simulink model "Magnetic_Levitation_Part3"  (R2022b)
settings: Solver=VariableStepAuto  StartTime=0.0  StopTime=10  RelTol=1e-3
settings Model: Creator=mhadi  LastModifiedBy=mhadi

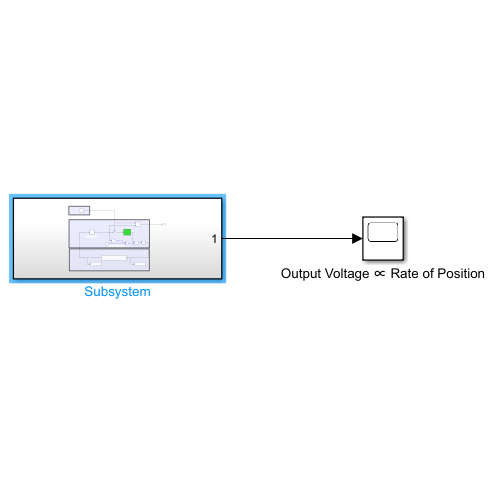
[thumbnail: Simulink's stored preview of the top-level diagram]
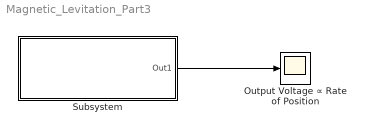
== system Magnetic_Levitation_Part3 ==
  Output Voltage ∝ Rate of Position : Scope
  Subsystem : Subsystem
  wires:
  Subsystem/1(Out1) -> Output Voltage ∝ Rate of Position/1

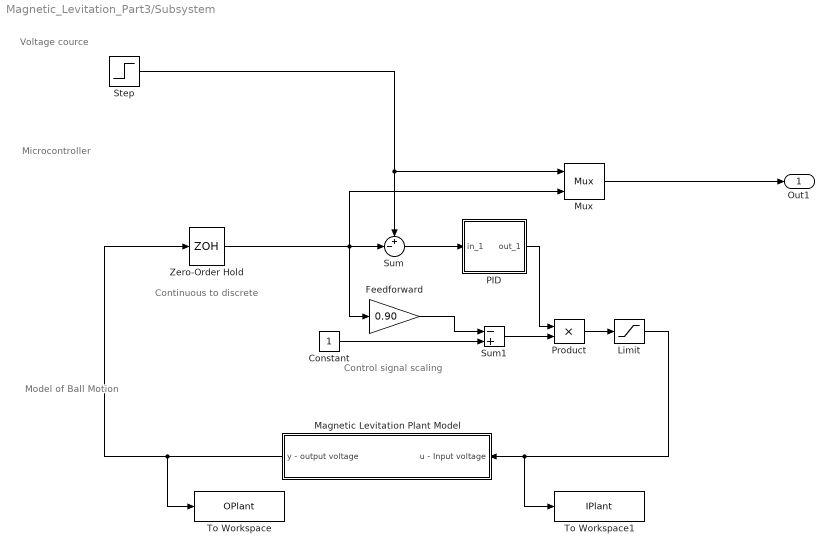
== system Magnetic_Levitation_Part3/Subsystem ==
  note: Voltage cource
  note: Model of Ball Motion
  note: Control signal scaling
  note: Continuous to discrete
  note: Microcontroller
  Constant : Constant  StatePerturbationForJacobian=1.0e-05
  Feedforward : Gain  StatePerturbationForJacobian=1.0e-05  Gain=0.90  SaturateOnIntegerOverflow=on  OutDataTypeStr=Inherit: Same as input  ParamDataTypeStr=Inherit: Same as input
  Limit : Saturate  StatePerturbationForJacobian=1.0e-05  UpperLimit=1  LowerLimit=0  ZeroCross=off
  Magnetic Levitation Plant Model : Subsystem  StatePerturbationForJacobian=1.0e-05
  Mux : Mux  StatePerturbationForJacobian=1.0e-05  Inputs=2
  PID : Subsystem  StatePerturbationForJacobian=1.0e-05  mask(PID){Kp=0.5, Ki=3, Kd=0, Ts=0.001}
      mask prompts: Ts "Sample time:"
      mask help: Discrete-time PID controller with limited integrator
      mask Display: disp('PID');
  Product : Product  StatePerturbationForJacobian=1.0e-05  InputSameDT=on  SaturateOnIntegerOverflow=on  OutDataTypeStr=Inherit: Same as first input
  Step : Step  StatePerturbationForJacobian=1.0e-05  Time=0  SampleTime=0
  Sum : Sum  StatePerturbationForJacobian=1.0e-05  Inputs=+-|  InputSameDT=on  SaturateOnIntegerOverflow=on  OutDataTypeStr=Inherit: Same as first input
  Sum1 : Sum  StatePerturbationForJacobian=1.0e-05  Inputs=-+  InputSameDT=on  SaturateOnIntegerOverflow=on  OutDataTypeStr=Inherit: Same as first input
  To Workspace : ToWorkspace  VariableName=OPlant  SaveFormat=Structure With Time  SampleTime=-1
      settings: Save2DSignal=2-D array (concatenate along first dimension)
  To Workspace1 : ToWorkspace  VariableName=IPlant  SaveFormat=Structure With Time  SampleTime=-1
      settings: Save2DSignal=2-D array (concatenate along first dimension)
  Zero-Order Hold : ZeroOrderHold  StatePerturbationForJacobian=1.0e-05  SampleTime=0.001
  Out1 : Outport
  wires:
  Limit/1 -> To Workspace1/1, Magnetic Levitation Plant Model/1(u - Input voltage)
  PID/1(out_1) -> Product/1
  Sum/1 -> PID/1(in_1)
  Feedforward/1 -> Sum1/1
  Mux/1 -> Out1/1
  Product/1 -> Limit/1
  Zero-Order Hold/1 -> Mux/2, Sum/2, Feedforward/1
  Magnetic Levitation Plant Model/1(y - output voltage) -> To Workspace/1, Zero-Order Hold/1
  Sum1/1 -> Product/2
  Constant/1 -> Sum1/2
  Step/1 -> Mux/1, Sum/1

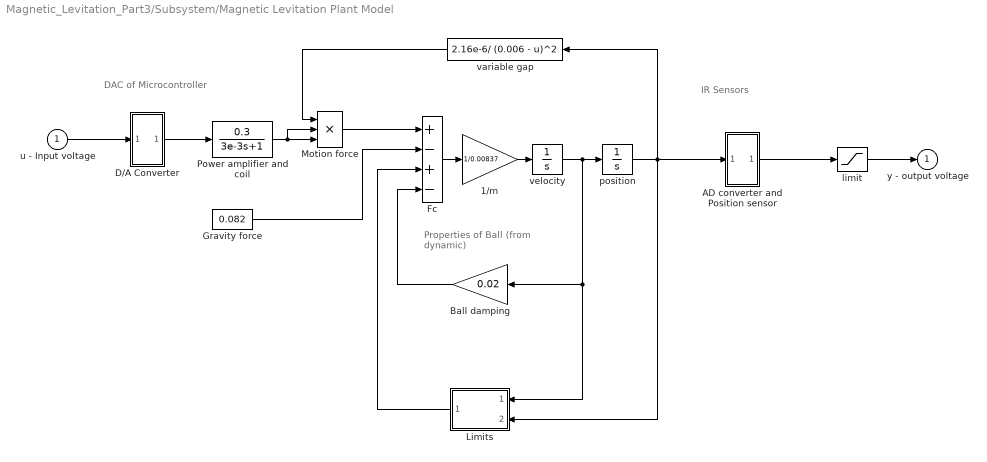
== system Magnetic_Levitation_Part3/Subsystem/Magnetic Levitation Plant Model ==
  note: Properties of Ball
      | (from dynamic)
  note: IR Sensors
  note: DAC of
      | Microcontroller
  u - Input voltage : Inport  StatePerturbationForJacobian=1.0e-05
  " limit" : Saturate  StatePerturbationForJacobian=1.0e-05  UpperLimit=0.998  LowerLimit=0  ZeroCross=off
  1/m : Gain  StatePerturbationForJacobian=1.0e-05  Gain=1/0.00837  SaturateOnIntegerOverflow=on  OutDataTypeStr=Inherit: Same as input  ParamDataTypeStr=Inherit: Same as input
  AD converter and Position sensor : Subsystem  StatePerturbationForJacobian=1.0e-05
      mask Display: disp('A/D')
  Ball damping : Gain  StatePerturbationForJacobian=1.0e-05  Gain=0.02  SaturateOnIntegerOverflow=on  OutDataTypeStr=Inherit: Same as input  ParamDataTypeStr=Inherit: Same as input
  D/A Converter : Subsystem  StatePerturbationForJacobian=1.0e-05
      mask Display: disp('D/A')
  Fc : Sum  StatePerturbationForJacobian=1.0e-05  Inputs=+-+-  InputSameDT=on  SaturateOnIntegerOverflow=on  OutDataTypeStr=Inherit: Same as first input
  Gravity force : Constant  StatePerturbationForJacobian=1.0e-05  Value=0.082
  Limits : Subsystem  StatePerturbationForJacobian=1.0e-05
      mask Display: disp('LIMIT')
  Motion force : Product  StatePerturbationForJacobian=1.0e-05  Inputs=3  InputSameDT=on  SaturateOnIntegerOverflow=on  OutDataTypeStr=Inherit: Same as first input
  Power amplifier and coil : TransferFcn  StatePerturbationForJacobian=1.0e-05  Numerator=[0.3]  Denominator=[3e-3 1]
  position : Integrator  StatePerturbationForJacobian=1.0e-05  LimitOutput=on  UpperSaturationLimit=0.005  LowerSaturationLimit=0  ZeroCross=off
  variable gap : Fcn  StatePerturbationForJacobian=1.0e-05  Expr=2.16e-6/ (0.006 - u)^2
  velocity : Integrator  StatePerturbationForJacobian=1.0e-05  ZeroCross=off
  y - output voltage : Outport  StatePerturbationForJacobian=1.0e-05
  wires:
  velocity/1 -> Ball damping/1, Limits/1(velocity), position/1
  Ball damping/1 -> Fc/4
  variable gap/1 -> Motion force/1
  1/m/1 -> velocity/1
  Fc/1 -> 1/m/1
  Motion force/1 -> Fc/1
  Gravity force/1 -> Fc/2
  D/A Converter/1(out_1) -> Power amplifier and coil/1
  u - Input voltage/1 -> D/A Converter/1(in_1)
  position/1 -> AD converter and Position sensor/1(in_1), variable gap/1, Limits/2(position)
  Limits/1(force) -> Fc/3
  Power amplifier and coil/1 -> Motion force/3, Motion force/2
  " limit"/1 -> y - output voltage/1
  AD converter and Position sensor/1(out_1) -> " limit"/1

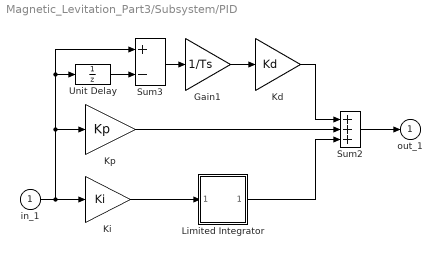
== system Magnetic_Levitation_Part3/Subsystem/PID ==
  in_1 : Inport  StatePerturbationForJacobian=1.0e-05
  Gain1 : Gain  StatePerturbationForJacobian=1.0e-05  Gain=1/Ts  SaturateOnIntegerOverflow=on  OutDataTypeStr=Inherit: Same as input  ParamDataTypeStr=Inherit: Same as input
  Kd : Gain  StatePerturbationForJacobian=1.0e-05  Gain=Kd  SaturateOnIntegerOverflow=on  OutDataTypeStr=Inherit: Same as input  ParamDataTypeStr=Inherit: Same as input
  Ki : Gain  StatePerturbationForJacobian=1.0e-05  Gain=Ki  SaturateOnIntegerOverflow=on  OutDataTypeStr=Inherit: Same as input  ParamDataTypeStr=Inherit: Same as input
  Kp : Gain  StatePerturbationForJacobian=1.0e-05  Gain=Kp  SaturateOnIntegerOverflow=on  OutDataTypeStr=Inherit: Same as input  ParamDataTypeStr=Inherit: Same as input
  Limited Integrator : Subsystem  StatePerturbationForJacobian=1.0e-05  mask(Discrete-Time Limited Integrator.){lower_limit=0, upper_limit=2, X0=0, Ts=Ts}
      mask prompts: lower_limit "Lower bound:"; upper_limit "Upper bound:"; X0 "Initial condition:"; Ts "Sampling Time:"
      mask help: Discrete-Time Limited Integrator.
      mask Help: Discrete-Time Limited Integrator. Unmask to see details.
      mask Display: plot(-1,-0.2,3.5,1.2,[0,1,2,2.9],[0,0,1,1],[0,1],[0.5,0.5], [.5,.5], [.8,.6], [.05,.35,.05,.35],[.4,.4,.2,.2], [.45,.65],[.3,.3], [.9,.9],[.2,.4]);
  Sum2 : Sum  StatePerturbationForJacobian=1.0e-05  Inputs=+++  InputSameDT=on  SaturateOnIntegerOverflow=on  OutDataTypeStr=Inherit: Same as first input
  Sum3 : Sum  StatePerturbationForJacobian=1.0e-05  Inputs=+-  InputSameDT=on  SaturateOnIntegerOverflow=on  OutDataTypeStr=Inherit: Same as first input
  Unit Delay : UnitDelay  StatePerturbationForJacobian=1.0e-05  SampleTime=Ts  HasFrameUpgradeWarning=on
  out_1 : Outport  StatePerturbationForJacobian=1.0e-05  InitialOutput=0
  wires:
  Unit Delay/1 -> Sum3/2
  Kd/1 -> Sum2/1
  Kp/1 -> Sum2/2
  Sum2/1 -> out_1/1
  Sum3/1 -> Gain1/1
  Gain1/1 -> Kd/1
  in_1/1 -> Ki/1, Sum3/1, Unit Delay/1, Kp/1
  Ki/1 -> Limited Integrator/1(in_1)
  Limited Integrator/1(out_1) -> Sum2/3

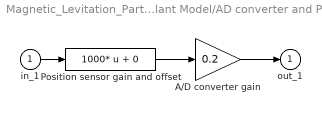
== system Magnetic_Levitation_Part3/Subsystem/Magnetic Levitation Plant Model/AD converter and Position sensor ==
  in_1 : Inport  StatePerturbationForJacobian=1.0e-05
  A/D converter gain : Gain  StatePerturbationForJacobian=1.0e-05  Gain=0.2  SaturateOnIntegerOverflow=on  OutDataTypeStr=Inherit: Same as input  ParamDataTypeStr=Inherit: Same as input
  Position sensor gain and offset : Fcn  StatePerturbationForJacobian=1.0e-05  Expr=1000* u + 0
  out_1 : Outport  StatePerturbationForJacobian=1.0e-05
  wires:
  in_1/1 -> Position sensor gain and offset/1
  Position sensor gain and offset/1 -> A/D converter gain/1
  A/D converter gain/1 -> out_1/1

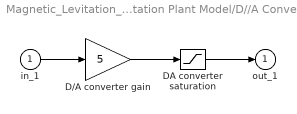
== system Magnetic_Levitation_Part3/Subsystem/Magnetic Levitation Plant Model/D//A Converter ==
  in_1 : Inport  StatePerturbationForJacobian=1.0e-05
  D/A converter gain : Gain  StatePerturbationForJacobian=1.0e-05  Gain=5  SaturateOnIntegerOverflow=on  OutDataTypeStr=Inherit: Same as input  ParamDataTypeStr=Inherit: Same as input
  DA converter saturation : Saturate  StatePerturbationForJacobian=1.0e-05  UpperLimit=5  LowerLimit=-5  ZeroCross=off
  out_1 : Outport  StatePerturbationForJacobian=1.0e-05
  wires:
  in_1/1 -> D/A converter gain/1
  DA converter saturation/1 -> out_1/1
  D/A converter gain/1 -> DA converter saturation/1

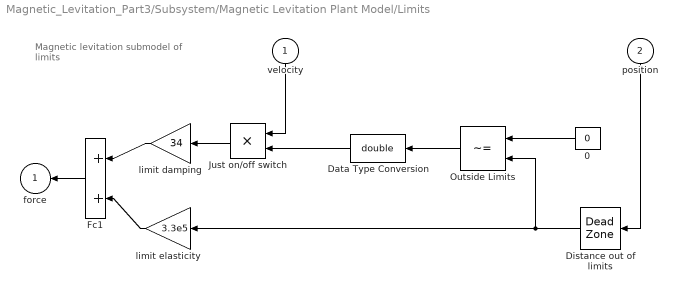
== system Magnetic_Levitation_Part3/Subsystem/Magnetic Levitation Plant Model/Limits ==
  note: Magnetic levitation
      | submodel of limits
  velocity : Inport  StatePerturbationForJacobian=1.0e-05
  position : Inport  StatePerturbationForJacobian=1.0e-05  Port=2
  0 : Constant  StatePerturbationForJacobian=1.0e-05  Value=0
  Data Type Conversion : DataTypeConversion  StatePerturbationForJacobian=1.0e-05  OutDataTypeStr=double
  Distance out of limits : DeadZone  StatePerturbationForJacobian=1.0e-05  LowerValue=0  UpperValue=0.005  ZeroCross=off
  Fc1 : Sum  StatePerturbationForJacobian=1.0e-05  InputSameDT=on  SaturateOnIntegerOverflow=on  OutDataTypeStr=Inherit: Same as first input
  "Just on/off switch " : Product  StatePerturbationForJacobian=1.0e-05  InputSameDT=on  SaturateOnIntegerOverflow=on  OutDataTypeStr=Inherit: Same as first input
  Outside Limits : RelationalOperator  StatePerturbationForJacobian=1.0e-05  Operator=~=
  limit damping : Gain  StatePerturbationForJacobian=1.0e-05  Gain=34  SaturateOnIntegerOverflow=on  OutDataTypeStr=Inherit: Same as input  ParamDataTypeStr=Inherit: Same as input
  limit elasticity : Gain  StatePerturbationForJacobian=1.0e-05  Gain=3.3e5  SaturateOnIntegerOverflow=on  OutDataTypeStr=Inherit: Same as input  ParamDataTypeStr=Inherit: Same as input
  force : Outport  StatePerturbationForJacobian=1.0e-05
  wires:
  Distance out of limits/1 -> Outside Limits/2, limit elasticity/1
  limit damping/1 -> Fc1/1
  limit elasticity/1 -> Fc1/2
  Outside Limits/1 -> Data Type Conversion/1
  0/1 -> Outside Limits/1
  "Just on/off switch "/1 -> limit damping/1
  velocity/1 -> "Just on/off switch "/1
  Fc1/1 -> force/1
  position/1 -> Distance out of limits/1
  Data Type Conversion/1 -> "Just on/off switch "/2

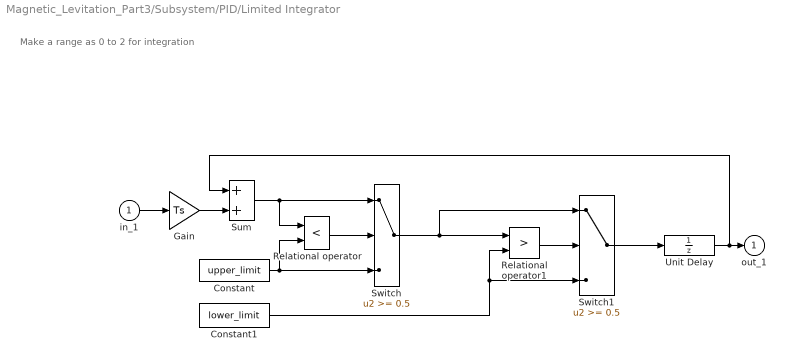
== system Magnetic_Levitation_Part3/Subsystem/PID/Limited Integrator ==
  note: Make a range as 0 to 2 for integration
  in_1 : Inport  StatePerturbationForJacobian=1.0e-05
  Constant : Constant  StatePerturbationForJacobian=1.0e-05  Value=upper_limit
  Constant1 : Constant  StatePerturbationForJacobian=1.0e-05  Value=lower_limit
  Gain : Gain  StatePerturbationForJacobian=1.0e-05  Gain=Ts  SaturateOnIntegerOverflow=on  OutDataTypeStr=Inherit: Same as input  ParamDataTypeStr=Inherit: Same as input
  Relational operator : RelationalOperator  StatePerturbationForJacobian=1.0e-05  Operator=<
  Relational operator1 : RelationalOperator  StatePerturbationForJacobian=1.0e-05  Operator=>
  Sum : Sum  StatePerturbationForJacobian=1.0e-05  InputSameDT=on  SaturateOnIntegerOverflow=on  OutDataTypeStr=Inherit: Same as first input
  Switch : Switch  StatePerturbationForJacobian=1.0e-05  Threshold=0.5  SaturateOnIntegerOverflow=off
  Switch1 : Switch  StatePerturbationForJacobian=1.0e-05  Threshold=0.5  SaturateOnIntegerOverflow=off
  Unit Delay : UnitDelay  StatePerturbationForJacobian=1.0e-05  InitialCondition=X0  SampleTime=Ts  HasFrameUpgradeWarning=on
  out_1 : Outport  StatePerturbationForJacobian=1.0e-05  InitialOutput=0
  wires:
  Unit Delay/1 -> out_1/1, Sum/1
  Switch1/1 -> Unit Delay/1
  Constant1/1 -> Relational operator1/2, Switch1/3
  Relational operator1/1 -> Switch1/2
  Switch/1 -> Relational operator1/1, Switch1/1
  Constant/1 -> Switch/3, Relational operator/2
  Gain/1 -> Sum/2
  Sum/1 -> Switch/1, Relational operator/1
  Relational operator/1 -> Switch/2
  in_1/1 -> Gain/1
